simulink model "Copy_of_ModeStatAndRsp"  (R2018b)
settings: Solver=FixedStepDiscrete  StartTime=0.0  StopTime=10.0  FixedStep=0.01  RelTol=1e-3
undefined symbols (not defined in the file): c_RecvL, c_RecvLR, c_RecvR, IfVeSMSeStNumConfig, KeSMSbMdChime2Enable_Val, KeSMSbSRSPosNumConfig_Val, KeSMSuChmReqDurnTm_Val, KeSMSuChmReqIntlTm_Val, KeSMSuRspStatHldTm_Val, MdRspLocal1, MdTp1, ModeNum, PowerMode1, SrcReqTp1, srsconvert
libraries: RspLib x47, simulink x1
(part 3 of 8)

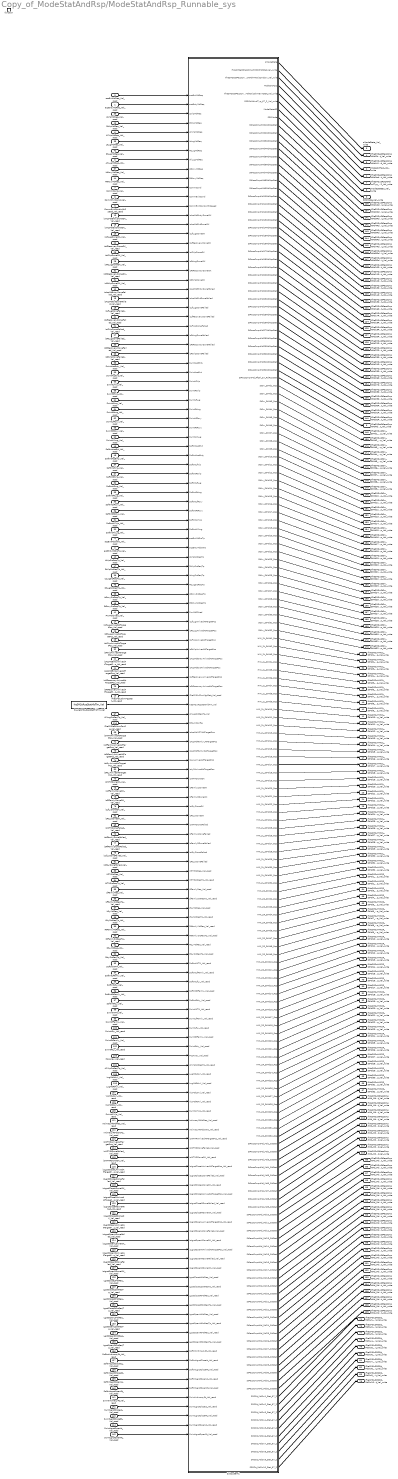
== system Copy_of_ModeStatAndRsp/ModeStatAndRsp_Runnable_sys ==
  acsEntyMdReq_Val_read : Inport
  acsEntyMdSrcTp_Val_read : Inport  Port=2
  acsExtMdReq_Val_read : Inport  Port=3
  acsExtMdSrcTp_Val_read : Inport  Port=4
  AllLugMdReq_Val_read : Inport  Port=5
  AllVipMdReq_Val_read : Inport  Port=6
  CommCond_Val_read : Inport  Port=7
  CommExitCond_Val_read : Inport  Port=8
  CommExitCondwithSpeed_Val_read : Inport  Port=9
  IfVeSMSuChmMgrStat_Val_read : Inport  Port=10
  isAcsMdEntryArrivedAtTargetPos_Val_read : Inport  Port=11
  isAcsMdEntryDoneFailed_Val_read : Inport  Port=12
  isAcsMdEntryDoneOK_Val_read : Inport  Port=13
  isAcsMdExtArrivedAtTargetPos_Val_read : Inport  Port=14
  isAcsMdExtDoneFailed_Val_read : Inport  Port=15
  isAcsMdExtDoneOK_Val_read : Inport  Port=16
  isLfLugArrivedAtTargetPos_Val_read : Inport  Port=17
  isLfLugDoneFailed_Val_read : Inport  Port=18
  isLfLugDoneOK_Val_read : Inport  Port=19
  isLfRecoveryArrivedAtTargetPos_Val_read : Inport  Port=20
  isLfRecoveryDoneFailed_Val_read : Inport  Port=21
  isLfRecoveryDoneOK_Val_read : Inport  Port=22
  isLfVipArrivedAtTargetPos_Val_read : Inport  Port=23
  isLfVipDoneFailed_Val_read : Inport  Port=24
  isLfVipDoneOK_Val_read : Inport  Port=25
  isRtLugArrivedAtTargetPos_Val_read : Inport  Port=26
  isRtLugDoneFailed_Val_read : Inport  Port=27
  isRtLugDoneOK_Val_read : Inport  Port=28
  isRtRecoveryArrivedAtTargetPos_Val_read : Inport  Port=29
  isRtRecoveryDoneFailed_Val_read : Inport  Port=30
  isRtRecoveryDoneOK_Val_read : Inport  Port=31
  isRtVipArrivedAtTargetPos_Val_read : Inport  Port=32
  isRtVipDoneFailed_Val_read : Inport  Port=33
  isRtVipDoneOK_Val_read : Inport  Port=34
  LtLugMdReq_Val_read : Inport  Port=35
  LtLugSrcReqTp_Val_read : Inport  Port=36
  LtRcvyMdReq_Val_read : Inport  Port=37
  LtRcvySrcReqTp_Val_read : Inport  Port=38
  LtVipMdReq_Val_read : Inport  Port=39
  LtVipSrcReqTp_Val_read : Inport  Port=40
  PwrMdChked_Val_read : Inport  Port=41
  RtLugMdReq_Val_read : Inport  Port=42
  RtLugSrcReqTp_Val_read : Inport  Port=43
  RtRcvyMdReq_Val_read : Inport  Port=44
  RtRcvySrcReqTp_Val_read : Inport  Port=45
  RtVipMdReq_Val_read : Inport  Port=46
  RtVipSrcReqTp_Val_read : Inport  Port=47
  SoftIntAcsEnty_Val_read : Inport  Port=48
  SoftIntAcsExt_Val_read : Inport  Port=49
  SoftIntAllLug_Val_read : Inport  Port=50
  SoftIntAllVip_Val_read : Inport  Port=51
  SoftIntLfLug_Val_read : Inport  Port=52
  SoftIntLfRcvy_Val_read : Inport  Port=53
  SoftIntLfVip_Val_read : Inport  Port=54
  SoftIntRtLug_Val_read : Inport  Port=55
  SoftIntRtRcvy_Val_read : Inport  Port=56
  SoftIntRtVip_Val_read : Inport  Port=57
  SwIntAcsEnty_Val_read : Inport  Port=58
  SwIntAcsExt_Val_read : Inport  Port=59
  SwIntAllLug_Val_read : Inport  Port=60
  SwIntLfLug_Val_read : Inport  Port=61
  SwIntLfRcvy_Val_read : Inport  Port=62
  SwIntLfVip_Val_read : Inport  Port=63
  SwIntRtLug_Val_read : Inport  Port=64
  SwIntRtRcvy_Val_read : Inport  Port=65
  SwIntRtVip_Val_read : Inport  Port=66
  AllLugSrcReqTp_Val_read : Inport  Port=67
  isINTMArrivedAtTargetPos_Val_read : Inport  Port=68
  isINTMDoneFailed_Val_read : Inport  Port=69
  isINTMDoneOK_Val_read : Inport  Port=70
  isLfFamlyArrivedAtTargetPos_Val_read : Inport  Port=71
  isLfFamlyDoneFailed_Val_read : Inport  Port=72
  isLfFamlyDoneOK_Val_read : Inport  Port=73
  isLfLyArrivedAtTargetPos_Val_read : Inport  Port=74
  isLfLyDoneFailed_Val_read : Inport  Port=75
  isLfLyDoneOK_Val_read : Inport  Port=76
  isRfFamlyDoneFailed_Val_read : Inport  Port=77
  isRfFamlyDoneOK_Val_read : Inport  Port=78
  isRtFamlyArrivedAtTargetPos_Val_read : Inport  Port=79
  isRtLyArrivedAtTargetPos_Val_read : Inport  Port=80
  isRtLyDoneFailed_Val_read : Inport  Port=81
  isRtLyDoneOK_Val_read : Inport  Port=82
  INTMMdReq_Val_read : Inport  Port=83
  INTMSrcReqTp_Val_read : Inport  Port=84
  LfFamlyReq_Val_read : Inport  Port=85
  LfFamlySrcReqTp_Val_read : Inport  Port=86
  LfLyMdReq_Val_read : Inport  Port=87
  LfLySrcReqTp_Val_read : Inport  Port=88
  RtFamlyMdReq_Val_read : Inport  Port=89
  RtFamlySrcReqTp_Val_read : Inport  Port=90
  RtLyMdReq_Val_read : Inport  Port=91
  RtLySrcReqTp_Val_read : Inport  Port=92
  SoftIntINTM_Val_read : Inport  Port=93
  SoftIntLfFamly_Val_read : Inport  Port=94
  SoftIntLfLy_Val_read : Inport  Port=95
  SoftIntRtFamly_Val_read : Inport  Port=96
  SoftIntRtLy_Val_read : Inport  Port=97
  SwIntINTM_Val_read : Inport  Port=98
  SwIntLfFamly_Val_read : Inport  Port=99
  SwIntLfLy_Val_read : Inport  Port=100
  SwIntRtFamly_Val_read : Inport  Port=101
  SwIntRtLy_Val_read : Inport  Port=102
  PosArray_Val_read : Inport  Port=103
  AllVipSrcReqTp_Val_read : Inport  Port=104
  LugMdLtAvl_Val_read : Inport  Port=105
  LugMdRtAvl_Val_read : Inport  Port=106
  VipMdLtAvl_Val_read : Inport  Port=107
  VipMdRtAvl_Val_read : Inport  Port=108
  SwIntAllVip_Val_read : Inport  Port=109
  IfVeSMSeStNumConfig_Val_read : Inport  Port=110
  IntimacyRtMdReq_Val_read : Inport  Port=111
  IntimacyRtMdSrcTp_Val_read : Inport  Port=112
  isINTMRArrivedAtTargetPos_Val_read : Inport  Port=113
  isINTMRDoneFailed_Val_read : Inport  Port=114
  isINTMRDoneOK_Val_read : Inport  Port=115
  isLgrstCloseLArrivedAtTargetPos_Val_read : Inport  Port=116
  isLgrstCloseLDoneFailed_Val_read : Inport  Port=117
  isLgrstCloseLDoneOK_Val_read : Inport  Port=118
  isLgrstCloseRArrivedAtTargetPos_Val_read : Inport  Port=119
  isLgrstCloseRDoneFailed_Val_read : Inport  Port=120
  isLgrstCloseRDoneOK_Val_read : Inport  Port=121
  isLgrstOpenLArrivedAtTargetPos_Val_read : Inport  Port=122
  isLgrstOpenLDoneFailed_Val_read : Inport  Port=123
  isLgrstOpenLDoneOK_Val_read : Inport  Port=124
  isLgrstOpenRArrivedAtTargetPos_Val_read : Inport  Port=125
  isLgrstOpenRDoneFailed_Val_read : Inport  Port=126
  isLgrstOpenRDoneOK_Val_read : Inport  Port=127
  LgrstCloseLtMdReq_Val_read : Inport  Port=128
  LgrstCloseLtSrcReqTp_Val_read : Inport  Port=129
  LgrstCloseRtMdReq_Val_read : Inport  Port=130
  LgrstCloseRtSrcReqTp_Val_read : Inport  Port=131
  LgrstOpenLtMdReq_Val_read : Inport  Port=132
  LgrstOpenLtSrcReqTp_Val_read : Inport  Port=133
  LgrstOpenRtMdReq_Val_read : Inport  Port=134
  LgrstOpenRtSrcReqTp_Val_read : Inport  Port=135
  SoftIntIntimacyRt_Val_read : Inport  Port=136
  SoftIntLgrstCloseLt_Val_read : Inport  Port=137
  SoftIntLgrstCloseRt_Val_read : Inport  Port=138
  SoftIntLgrstOpenLt_Val_read : Inport  Port=139
  SoftIntLgrstOpenRt_Val_read : Inport  Port=140
  SwIntIntimacyRt_Val_read : Inport  Port=141
  SwIntLgrstCloseLt_Val_read : Inport  Port=142
  SwIntLgrstCloseRt_Val_read : Inport  Port=143
  SwIntLgrstOpenLt_Val_read : Inport  Port=144
  SwIntLgrstOpenRt_Val_read : Inport  Port=145
  function : TriggerPort  TriggerType=function-call  VariantControl=(inherit)  SampleTimeType=periodic  SampleTime=-1
  PA_KeSMSuRspStatHldTm_Val : Constant  Value=KeSMSuRspStatHldTm_Val
  Subsystem1 : Subsystem
  IfVeSMSeStPassCmprtMdNoti2ChmEvntStat_Val_write : Outport
      settings: EnsureOutportIsVirtual=on
  ModeSrcTpLt_Val_write : Outport  Port=2
      settings: EnsureOutportIsVirtual=on
  oModeState_Val_write : Outport  Port=3
      settings: EnsureOutportIsVirtual=on
  IfVeSMSeStPassCmprtMdCrtMdStat_Val_write : Outport  Port=4
      settings: EnsureOutportIsVirtual=on
  IfVeSMSuStPassCmprtMdHMIDisCmd_Val_write : Outport  Port=5
      settings: EnsureOutportIsVirtual=on
  IfVeSMSeStPassCmprtMdRclRspStat_Val_write : Outport  Port=6
      settings: EnsureOutportIsVirtual=on
  IfVeSMSuSRSCrtMdIndTyp_67_2_Val_write : Outport  Port=7
      settings: EnsureOutportIsVirtual=on
  modestate32_Val_write : Outport  Port=8
      settings: EnsureOutportIsVirtual=on
  SRSMode_Val_write : Outport  Port=9
      settings: EnsureOutportIsVirtual=on
  IfVeSMSuHMI2L_StMd1_Rsp_Val_write : Outport  Port=10
      settings: EnsureOutportIsVirtual=on
  IfVeSMSuHMI2L_StMd10_Rsp_Val_write : Outport  Port=11
      settings: EnsureOutportIsVirtual=on
  IfVeSMSuHMI2L_StMd11_Rsp_Val_write : Outport  Port=12
      settings: EnsureOutportIsVirtual=on
  IfVeSMSuHMI2L_StMd12_Rsp_Val_write : Outport  Port=13
      settings: EnsureOutportIsVirtual=on
  IfVeSMSuHMI2L_StMd13_Rsp_Val_write : Outport  Port=14
      settings: EnsureOutportIsVirtual=on
  IfVeSMSuHMI2L_StMd14_Rsp_Val_write : Outport  Port=15
      settings: EnsureOutportIsVirtual=on
  IfVeSMSuHMI2L_StMd15_Rsp_Val_write : Outport  Port=16
      settings: EnsureOutportIsVirtual=on
  IfVeSMSuHMI2L_StMd16_Rsp_Val_write : Outport  Port=17
      settings: EnsureOutportIsVirtual=on
  IfVeSMSuHMI2L_StMd17_Rsp_Val_write : Outport  Port=18
      settings: EnsureOutportIsVirtual=on
  IfVeSMSuHMI2L_StMd18_Rsp_Val_write : Outport  Port=19
      settings: EnsureOutportIsVirtual=on
  IfVeSMSuHMI2L_StMd19_Rsp_Val_write : Outport  Port=20
      settings: EnsureOutportIsVirtual=on
  IfVeSMSuHMI2L_StMd2_Rsp_Val_write : Outport  Port=21
      settings: EnsureOutportIsVirtual=on
  IfVeSMSuHMI2L_StMd20_Rsp_Val_write : Outport  Port=22
      settings: EnsureOutportIsVirtual=on
  IfVeSMSuHMI2L_StMd21_Rsp_Val_write : Outport  Port=23
      settings: EnsureOutportIsVirtual=on
  IfVeSMSuHMI2L_StMd22_Rsp_Val_write : Outport  Port=24
      settings: EnsureOutportIsVirtual=on
  IfVeSMSuHMI2L_StMd23_Rsp_Val_write : Outport  Port=25
      settings: EnsureOutportIsVirtual=on
  IfVeSMSuHMI2L_StMd24_Rsp_Val_write : Outport  Port=26
      settings: EnsureOutportIsVirtual=on
  IfVeSMSuHMI2L_StMd25_Rsp_Val_write : Outport  Port=27
      settings: EnsureOutportIsVirtual=on
  IfVeSMSuHMI2L_StMd26_Rsp_Val_write : Outport  Port=28
      settings: EnsureOutportIsVirtual=on
  IfVeSMSuHMI2L_StMd27_Rsp_Val_write : Outport  Port=29
      settings: EnsureOutportIsVirtual=on
  IfVeSMSuHMI2L_StMd28_Rsp_Val_write : Outport  Port=30
      settings: EnsureOutportIsVirtual=on
  IfVeSMSuHMI2L_StMd29_Rsp_Val_write : Outport  Port=31
      settings: EnsureOutportIsVirtual=on
  IfVeSMSuHMI2L_StMd3_Rsp_Val_write : Outport  Port=32
      settings: EnsureOutportIsVirtual=on
  IfVeSMSuHMI2L_StMd30_Rsp_Val_write : Outport  Port=33
      settings: EnsureOutportIsVirtual=on
  IfVeSMSuHMI2L_StMd31_Rsp_Val_write : Outport  Port=34
      settings: EnsureOutportIsVirtual=on
  IfVeSMSuHMI2L_StMd32_Rsp_Val_write : Outport  Port=35
      settings: EnsureOutportIsVirtual=on
  IfVeSMSuHMI2L_StMd4_Rsp_Val_write : Outport  Port=36
      settings: EnsureOutportIsVirtual=on
  IfVeSMSuHMI2L_StMd5_Rsp_Val_write : Outport  Port=37
      settings: EnsureOutportIsVirtual=on
  IfVeSMSuHMI2L_StMd6_Rsp_Val_write : Outport  Port=38
      settings: EnsureOutportIsVirtual=on
  IfVeSMSuHMI2L_StMd7_Rsp_Val_write : Outport  Port=39
      settings: EnsureOutportIsVirtual=on
  IfVeSMSuHMI2L_StMd8_Rsp_Val_write : Outport  Port=40
      settings: EnsureOutportIsVirtual=on
  IfVeSMSuHMI2L_StMd9_Rsp_Val_write : Outport  Port=41
      settings: EnsureOutportIsVirtual=on
  IfVeSMSuHMI2R_StMd1_Rsp_Val_write : Outport  Port=42
      settings: EnsureOutportIsVirtual=on
  IfVeSMSuHMI2R_StMd10_Rsp_Val_write : Outport  Port=43
      settings: EnsureOutportIsVirtual=on
  IfVeSMSuHMI2R_StMd11_Rsp_Val_write : Outport  Port=44
      settings: EnsureOutportIsVirtual=on
  IfVeSMSuHMI2R_StMd12_Rsp_Val_write : Outport  Port=45
      settings: EnsureOutportIsVirtual=on
  IfVeSMSuHMI2R_StMd13_Rsp_Val_write : Outport  Port=46
      settings: EnsureOutportIsVirtual=on
  IfVeSMSuHMI2R_StMd14_Rsp_Val_write : Outport  Port=47
      settings: EnsureOutportIsVirtual=on
  IfVeSMSuHMI2R_StMd15_Rsp_Val_write : Outport  Port=48
      settings: EnsureOutportIsVirtual=on
  IfVeSMSuHMI2R_StMd16_Rsp_Val_write : Outport  Port=49
      settings: EnsureOutportIsVirtual=on
  IfVeSMSuHMI2R_StMd17_Rsp_Val_write : Outport  Port=50
      settings: EnsureOutportIsVirtual=on
  IfVeSMSuHMI2R_StMd18_Rsp_Val_write : Outport  Port=51
      settings: EnsureOutportIsVirtual=on
  IfVeSMSuHMI2R_StMd19_Rsp_Val_write : Outport  Port=52
      settings: EnsureOutportIsVirtual=on
  IfVeSMSuHMI2R_StMd2_Rsp_Val_write : Outport  Port=53
      settings: EnsureOutportIsVirtual=on
  IfVeSMSuHMI2R_StMd20_Rsp_Val_write : Outport  Port=54
      settings: EnsureOutportIsVirtual=on
  IfVeSMSuHMI2R_StMd21_Rsp_Val_write : Outport  Port=55
      settings: EnsureOutportIsVirtual=on
  IfVeSMSuHMI2R_StMd22_Rsp_Val_write : Outport  Port=56
      settings: EnsureOutportIsVirtual=on
  IfVeSMSuHMI2R_StMd23_Rsp_Val_write : Outport  Port=57
      settings: EnsureOutportIsVirtual=on
  IfVeSMSuHMI2R_StMd24_Rsp_Val_write : Outport  Port=58
      settings: EnsureOutportIsVirtual=on
  IfVeSMSuHMI2R_StMd25_Rsp_Val_write : Outport  Port=59
      settings: EnsureOutportIsVirtual=on
  IfVeSMSuHMI2R_StMd26_Rsp_Val_write : Outport  Port=60
      settings: EnsureOutportIsVirtual=on
  IfVeSMSuHMI2R_StMd27_Rsp_Val_write : Outport  Port=61
      settings: EnsureOutportIsVirtual=on
  IfVeSMSuHMI2R_StMd28_Rsp_Val_write : Outport  Port=62
      settings: EnsureOutportIsVirtual=on
  IfVeSMSuHMI2R_StMd29_Rsp_Val_write : Outport  Port=63
      settings: EnsureOutportIsVirtual=on
  IfVeSMSuHMI2R_StMd3_Rsp_Val_write : Outport  Port=64
      settings: EnsureOutportIsVirtual=on
  IfVeSMSuHMI2R_StMd30_Rsp_Val_write : Outport  Port=65
      settings: EnsureOutportIsVirtual=on
  IfVeSMSuHMI2R_StMd31_Rsp_Val_write : Outport  Port=66
      settings: EnsureOutportIsVirtual=on
  IfVeSMSuHMI2R_StMd32_Rsp_Val_write : Outport  Port=67
      settings: EnsureOutportIsVirtual=on
  IfVeSMSuHMI2R_StMd4_Rsp_Val_write : Outport  Port=68
      settings: EnsureOutportIsVirtual=on
  IfVeSMSuHMI2R_StMd5_Rsp_Val_write : Outport  Port=69
      settings: EnsureOutportIsVirtual=on
  IfVeSMSuHMI2R_StMd6_Rsp_Val_write : Outport  Port=70
      settings: EnsureOutportIsVirtual=on
  IfVeSMSuHMI2R_StMd7_Rsp_Val_write : Outport  Port=71
      settings: EnsureOutportIsVirtual=on
  IfVeSMSuHMI2R_StMd8_Rsp_Val_write : Outport  Port=72
      settings: EnsureOutportIsVirtual=on
  IfVeSMSuHMI2R_StMd9_Rsp_Val_write : Outport  Port=73
      settings: EnsureOutportIsVirtual=on
  IfVeSMSuSRSCrt_MdSw1_Stat_Val_write : Outport  Port=74
      settings: EnsureOutportIsVirtual=on
  IfVeSMSuSRSCrt_MdSw10_Stat_Val_write : Outport  Port=75
      settings: EnsureOutportIsVirtual=on
  IfVeSMSuSRSCrt_MdSw2_Stat_Val_write : Outport  Port=76
      settings: EnsureOutportIsVirtual=on
  IfVeSMSuSRSCrt_MdSw3_Stat_Val_write : Outport  Port=77
      settings: EnsureOutportIsVirtual=on
  IfVeSMSuSRSCrt_MdSw4_Stat_Val_write : Outport  Port=78
      settings: EnsureOutportIsVirtual=on
  IfVeSMSuSRSCrt_MdSw5_Stat_Val_write : Outport  Port=79
      settings: EnsureOutportIsVirtual=on
  IfVeSMSuSRSCrt_MdSw6_Stat_Val_write : Outport  Port=80
      settings: EnsureOutportIsVirtual=on
  IfVeSMSuSRSCrt_MdSw7_Stat_Val_write : Outport  Port=81
      settings: EnsureOutportIsVirtual=on
  IfVeSMSuSRSCrt_MdSw8_Stat_Val_write : Outport  Port=82
      settings: EnsureOutportIsVirtual=on
  IfVeSMSuSRSCrt_MdSw9_Stat_Val_write : Outport  Port=83
      settings: EnsureOutportIsVirtual=on
  IfVeSMSuStPassCmprtMd_Md1_CrtStat_Val_write : Outport  Port=84
      settings: EnsureOutportIsVirtual=on
  IfVeSMSuStPassCmprtMd_Md10_CrtStat_Val_write : Outport  Port=85
      settings: EnsureOutportIsVirtual=on
  IfVeSMSuStPassCmprtMd_Md11_CrtStat_Val_write : Outport  Port=86
      settings: EnsureOutportIsVirtual=on
  IfVeSMSuStPassCmprtMd_Md12_CrtStat_Val_write : Outport  Port=87
      settings: EnsureOutportIsVirtual=on
  IfVeSMSuStPassCmprtMd_Md13_CrtStat_Val_write : Outport  Port=88
      settings: EnsureOutportIsVirtual=on
  IfVeSMSuStPassCmprtMd_Md14_CrtStat_Val_write : Outport  Port=89
      settings: EnsureOutportIsVirtual=on
  IfVeSMSuStPassCmprtMd_Md15_CrtStat_Val_write : Outport  Port=90
      settings: EnsureOutportIsVirtual=on
  IfVeSMSuStPassCmprtMd_Md16_CrtStat_Val_write : Outport  Port=91
      settings: EnsureOutportIsVirtual=on
  IfVeSMSuStPassCmprtMd_Md17_CrtStat_Val_write : Outport  Port=92
      settings: EnsureOutportIsVirtual=on
  IfVeSMSuStPassCmprtMd_Md18_CrtStat_Val_write : Outport  Port=93
      settings: EnsureOutportIsVirtual=on
  IfVeSMSuStPassCmprtMd_Md19_CrtStat_Val_write : Outport  Port=94
      settings: EnsureOutportIsVirtual=on
  IfVeSMSuStPassCmprtMd_Md2_CrtStat_Val_write : Outport  Port=95
      settings: EnsureOutportIsVirtual=on
  IfVeSMSuStPassCmprtMd_Md20_CrtStat_Val_write : Outport  Port=96
      settings: EnsureOutportIsVirtual=on
  IfVeSMSuStPassCmprtMd_Md21_CrtStat_Val_write : Outport  Port=97
      settings: EnsureOutportIsVirtual=on
  IfVeSMSuStPassCmprtMd_Md22_CrtStat_Val_write : Outport  Port=98
      settings: EnsureOutportIsVirtual=on
  IfVeSMSuStPassCmprtMd_Md23_CrtStat_Val_write : Outport  Port=99
      settings: EnsureOutportIsVirtual=on
  IfVeSMSuStPassCmprtMd_Md24_CrtStat_Val_write : Outport  Port=100
      settings: EnsureOutportIsVirtual=on
  IfVeSMSuStPassCmprtMd_Md25_CrtStat_Val_write : Outport  Port=101
      settings: EnsureOutportIsVirtual=on
  IfVeSMSuStPassCmprtMd_Md26_CrtStat_Val_write : Outport  Port=102
      settings: EnsureOutportIsVirtual=on
  IfVeSMSuStPassCmprtMd_Md27_CrtStat_Val_write : Outport  Port=103
      settings: EnsureOutportIsVirtual=on
  IfVeSMSuStPassCmprtMd_Md28_CrtStat_Val_write : Outport  Port=104
      settings: EnsureOutportIsVirtual=on
  IfVeSMSuStPassCmprtMd_Md29_CrtStat_Val_write : Outport  Port=105
      settings: EnsureOutportIsVirtual=on
  IfVeSMSuStPassCmprtMd_Md3_CrtStat_Val_write : Outport  Port=106
      settings: EnsureOutportIsVirtual=on
  IfVeSMSuStPassCmprtMd_Md30_CrtStat_Val_write : Outport  Port=107
      settings: EnsureOutportIsVirtual=on
  IfVeSMSuStPassCmprtMd_Md31_CrtStat_Val_write : Outport  Port=108
      settings: EnsureOutportIsVirtual=on
  IfVeSMSuStPassCmprtMd_Md32_CrtStat_Val_write : Outport  Port=109
      settings: EnsureOutportIsVirtual=on
  IfVeSMSuStPassCmprtMd_Md4_CrtStat_Val_write : Outport  Port=110
      settings: EnsureOutportIsVirtual=on
  IfVeSMSuStPassCmprtMd_Md5_CrtStat_Val_write : Outport  Port=111
      settings: EnsureOutportIsVirtual=on
  IfVeSMSuStPassCmprtMd_Md6_CrtStat_Val_write : Outport  Port=112
      settings: EnsureOutportIsVirtual=on
  IfVeSMSuStPassCmprtMd_Md7_CrtStat_Val_write : Outport  Port=113
      settings: EnsureOutportIsVirtual=on
  IfVeSMSuStPassCmprtMd_Md8_CrtStat_Val_write : Outport  Port=114
      settings: EnsureOutportIsVirtual=on
  IfVeSMSuStPassCmprtMd_Md9_CrtStat_Val_write : Outport  Port=115
      settings: EnsureOutportIsVirtual=on
  IfVeSMSuStPassCmprtMd10RclRspStat_Val_write : Outport  Port=116
      settings: EnsureOutportIsVirtual=on
  IfVeSMSuStPassCmprtMd11RclRspStat_Val_write : Outport  Port=117
      settings: EnsureOutportIsVirtual=on
  IfVeSMSuStPassCmprtMd12RclRspStat_Val_write : Outport  Port=118
      settings: EnsureOutportIsVirtual=on
  IfVeSMSuStPassCmprtMd13RclRspStat_Val_write : Outport  Port=119
      settings: EnsureOutportIsVirtual=on
  IfVeSMSuStPassCmprtMd14RclRspStat_Val_write : Outport  Port=120
      settings: EnsureOutportIsVirtual=on
  IfVeSMSuStPassCmprtMd15RclRspStat_Val_write : Outport  Port=121
      settings: EnsureOutportIsVirtual=on
  IfVeSMSuStPassCmprtMd16RclRspStat_Val_write : Outport  Port=122
      settings: EnsureOutportIsVirtual=on
  IfVeSMSuStPassCmprtMd17RclRspStat_Val_write : Outport  Port=123
      settings: EnsureOutportIsVirtual=on
  IfVeSMSuStPassCmprtMd18RclRspStat_Val_write : Outport  Port=124
      settings: EnsureOutportIsVirtual=on
  IfVeSMSuStPassCmprtMd19RclRspStat_Val_write : Outport  Port=125
      settings: EnsureOutportIsVirtual=on
  IfVeSMSuStPassCmprtMd1RclRspStat_Val_write : Outport  Port=126
      settings: EnsureOutportIsVirtual=on
  IfVeSMSuStPassCmprtMd20RclRspStat_Val_write : Outport  Port=127
      settings: EnsureOutportIsVirtual=on
  IfVeSMSuStPassCmprtMd21RclRspStat_Val_write : Outport  Port=128
      settings: EnsureOutportIsVirtual=on
  IfVeSMSuStPassCmprtMd22RclRspStat_Val_write : Outport  Port=129
      settings: EnsureOutportIsVirtual=on
  IfVeSMSuStPassCmprtMd23RclRspStat_Val_write : Outport  Port=130
      settings: EnsureOutportIsVirtual=on
  IfVeSMSuStPassCmprtMd24RclRspStat_Val_write : Outport  Port=131
      settings: EnsureOutportIsVirtual=on
  IfVeSMSuStPassCmprtMd25RclRspStat_Val_write : Outport  Port=132
      settings: EnsureOutportIsVirtual=on
  IfVeSMSuStPassCmprtMd26RclRspStat_Val_write : Outport  Port=133
      settings: EnsureOutportIsVirtual=on
  IfVeSMSuStPassCmprtMd27RclRspStat_Val_write : Outport  Port=134
      settings: EnsureOutportIsVirtual=on
  IfVeSMSuStPassCmprtMd28RclRspStat_Val_write : Outport  Port=135
      settings: EnsureOutportIsVirtual=on
  IfVeSMSuStPassCmprtMd29RclRspStat_Val_write : Outport  Port=136
      settings: EnsureOutportIsVirtual=on
  IfVeSMSuStPassCmprtMd2RclRspStat_Val_write : Outport  Port=137
      settings: EnsureOutportIsVirtual=on
  IfVeSMSuStPassCmprtMd30RclRspStat_Val_write : Outport  Port=138
      settings: EnsureOutportIsVirtual=on
  IfVeSMSuStPassCmprtMd31RclRspStat_Val_write : Outport  Port=139
      settings: EnsureOutportIsVirtual=on
  IfVeSMSuStPassCmprtMd32RclRspStat_Val_write : Outport  Port=140
      settings: EnsureOutportIsVirtual=on
  IfVeSMSuStPassCmprtMd3RclRspStat_Val_write : Outport  Port=141
      settings: EnsureOutportIsVirtual=on
  IfVeSMSuStPassCmprtMd4RclRspStat_Val_write : Outport  Port=142
      settings: EnsureOutportIsVirtual=on
  IfVeSMSuStPassCmprtMd5RclRspStat_Val_write : Outport  Port=143
      settings: EnsureOutportIsVirtual=on
  IfVeSMSuStPassCmprtMd6RclRspStat_Val_write : Outport  Port=144
      settings: EnsureOutportIsVirtual=on
  IfVeSMSuStPassCmprtMd7RclRspStat_Val_write : Outport  Port=145
      settings: EnsureOutportIsVirtual=on
  IfVeSMSuStPassCmprtMd8RclRspStat_Val_write : Outport  Port=146
      settings: EnsureOutportIsVirtual=on
  IfVeSMSuStPassCmprtMd9RclRspStat_Val_write : Outport  Port=147
      settings: EnsureOutportIsVirtual=on
  IfVeSMSuStSrv_StMd1_Rsp_Val_write : Outport  Port=148
      settings: EnsureOutportIsVirtual=on
  IfVeSMSuStSrv_StMd10_Rsp_Val_write : Outport  Port=149
      settings: EnsureOutportIsVirtual=on
  IfVeSMSuStSrv_StMd11_Rsp_Val_write : Outport  Port=150
      settings: EnsureOutportIsVirtual=on
  IfVeSMSuStSrv_StMd12_Rsp_Val_write : Outport  Port=151
      settings: EnsureOutportIsVirtual=on
  IfVeSMSuStSrv_StMd13_Rsp_Val_write : Outport  Port=152
      settings: EnsureOutportIsVirtual=on
  IfVeSMSuStSrv_StMd14_Rsp_Val_write : Outport  Port=153
      settings: EnsureOutportIsVirtual=on
  IfVeSMSuStSrv_StMd15_Rsp_Val_write : Outport  Port=154
      settings: EnsureOutportIsVirtual=on
  IfVeSMSuStSrv_StMd16_Rsp_Val_write : Outport  Port=155
      settings: EnsureOutportIsVirtual=on
  IfVeSMSuStSrv_StMd17_Rsp_Val_write : Outport  Port=156
      settings: EnsureOutportIsVirtual=on
  IfVeSMSuStSrv_StMd18_Rsp_Val_write : Outport  Port=157
      settings: EnsureOutportIsVirtual=on
  IfVeSMSuStSrv_StMd19_Rsp_Val_write : Outport  Port=158
      settings: EnsureOutportIsVirtual=on
  IfVeSMSuStSrv_StMd2_Rsp_Val_write : Outport  Port=159
      settings: EnsureOutportIsVirtual=on
  IfVeSMSuStSrv_StMd20_Rsp_Val_write : Outport  Port=160
      settings: EnsureOutportIsVirtual=on
  IfVeSMSuStSrv_StMd21_Rsp_Val_write : Outport  Port=161
      settings: EnsureOutportIsVirtual=on
  IfVeSMSuStSrv_StMd22_Rsp_Val_write : Outport  Port=162
      settings: EnsureOutportIsVirtual=on
  IfVeSMSuStSrv_StMd23_Rsp_Val_write : Outport  Port=163
      settings: EnsureOutportIsVirtual=on
  IfVeSMSuStSrv_StMd24_Rsp_Val_write : Outport  Port=164
      settings: EnsureOutportIsVirtual=on
  IfVeSMSuStSrv_StMd25_Rsp_Val_write : Outport  Port=165
      settings: EnsureOutportIsVirtual=on
  IfVeSMSuStSrv_StMd26_Rsp_Val_write : Outport  Port=166
      settings: EnsureOutportIsVirtual=on
  IfVeSMSuStSrv_StMd27_Rsp_Val_write : Outport  Port=167
      settings: EnsureOutportIsVirtual=on
  IfVeSMSuStSrv_StMd28_Rsp_Val_write : Outport  Port=168
      settings: EnsureOutportIsVirtual=on
  IfVeSMSuStSrv_StMd29_Rsp_Val_write : Outport  Port=169
      settings: EnsureOutportIsVirtual=on
  IfVeSMSuStSrv_StMd3_Rsp_Val_write : Outport  Port=170
      settings: EnsureOutportIsVirtual=on
  IfVeSMSuStSrv_StMd30_Rsp_Val_write : Outport  Port=171
      settings: EnsureOutportIsVirtual=on
  IfVeSMSuStSrv_StMd31_Rsp_Val_write : Outport  Port=172
      settings: EnsureOutportIsVirtual=on
  IfVeSMSuStSrv_StMd32_Rsp_Val_write : Outport  Port=173
      settings: EnsureOutportIsVirtual=on
  IfVeSMSuStSrv_StMd4_Rsp_Val_write : Outport  Port=174
      settings: EnsureOutportIsVirtual=on
  IfVeSMSuStSrv_StMd5_Rsp_Val_write : Outport  Port=175
      settings: EnsureOutportIsVirtual=on
  IfVeSMSuStSrv_StMd6_Rsp_Val_write : Outport  Port=176
      settings: EnsureOutportIsVirtual=on
  IfVeSMSuStSrv_StMd7_Rsp_Val_write : Outport  Port=177
      settings: EnsureOutportIsVirtual=on
  IfVeSMSuStSrv_StMd8_Rsp_Val_write : Outport  Port=178
      settings: EnsureOutportIsVirtual=on
  IfVeSMSuStSrv_StMd9_Rsp_Val_write : Outport  Port=179
      settings: EnsureOutportIsVirtual=on
  wires:
  acsEntyMdSrcTp_Val_read/1 -> Subsystem1/50(acsEntyMdSrcTp)
  acsExtMdReq_Val_read/1 -> Subsystem1/1(acsExtMdReq)
  acsExtMdSrcTp_Val_read/1 -> Subsystem1/49(acsExtMdSrcTp)
  AllLugMdReq_Val_read/1 -> Subsystem1/8(AllLugMdReq)
  AllVipMdReq_Val_read/1 -> Subsystem1/5(AllVipMdReq)
  CommCond_Val_read/1 -> Subsystem1/11(CommCond)
  CommExitCond_Val_read/1 -> Subsystem1/12(CommExitCond)
  CommExitCondwithSpeed_Val_read/1 -> Subsystem1/13(CommExitCondwithSpeed)
  IfVeSMSuChmMgrStat_Val_read/1 -> Subsystem1/66(IfVeSMSuChmMgrStat_Val_read)
  isAcsMdEntryArrivedAtTargetPos_Val_read/1 -> Subsystem1/62(isAcsMdEntryArrivedAtTargetPos)
  isAcsMdEntryDoneFailed_Val_read/1 -> Subsystem1/22(isAcsMdEntryDoneFailed)
  isAcsMdEntryDoneOK_Val_read/1 -> Subsystem1/14(isAcsMdEntryDoneOK)
  isAcsMdExtArrivedAtTargetPos_Val_read/1 -> Subsystem1/63(isAcsMdExtArrivedAtTargetPos)
  isAcsMdExtDoneFailed_Val_read/1 -> Subsystem1/23(isAcsMdExtDoneFailed)
  isAcsMdExtDoneOK_Val_read/1 -> Subsystem1/15(isAcsMdExtDoneOK)
  isLfLugDoneFailed_Val_read/1 -> Subsystem1/24(isLfLugDoneFailed)
  isLfLugDoneOK_Val_read/1 -> Subsystem1/16(isLfLugDoneOK)
  isLfRecoveryArrivedAtTargetPos_Val_read/1 -> Subsystem1/64(isLfRecoveryArrivedAtTargetPos)
  isLfRecoveryDoneFailed_Val_read/1 -> Subsystem1/25(isLfRecoveryDoneFailed)
  isLfRecoveryDoneOK_Val_read/1 -> Subsystem1/17(isLfRecoveryDoneOK)
  isLfVipArrivedAtTargetPos_Val_read/1 -> Subsystem1/60(isLfVipArrivedAtTargetPos)
  isLfVipDoneFailed_Val_read/1 -> Subsystem1/26(isLfVipDoneFailed)
  isLfVipDoneOK_Val_read/1 -> Subsystem1/18(isLfVipDoneOK)
  isRtLugArrivedAtTargetPos_Val_read/1 -> Subsystem1/59(isRtLugArrivedAtTargetPos)
  isRtLugDoneFailed_Val_read/1 -> Subsystem1/27(isRtLugDoneFailed)
  isRtLugDoneOK_Val_read/1 -> Subsystem1/19(isRtLugDoneOK)
  isRtRecoveryArrivedAtTargetPos_Val_read/1 -> Subsystem1/65(isRtRecoveryArrivedAtTargetPos)
  isRtRecoveryDoneFailed_Val_read/1 -> Subsystem1/28(isRtRecoveryDoneFailed)
  isRtRecoveryDoneOK_Val_read/1 -> Subsystem1/20(isRtRecoveryDoneOK)
  isRtVipArrivedAtTargetPos_Val_read/1 -> Subsystem1/61(isRtVipArrivedAtTargetPos)
  isRtVipDoneFailed_Val_read/1 -> Subsystem1/29(isRtVipDoneFailed)
  isRtVipDoneOK_Val_read/1 -> Subsystem1/21(isRtVipDoneOK)
  LtLugMdReq_Val_read/1 -> Subsystem1/6(LtLugMdReq)
  LtLugSrcReqTp_Val_read/1 -> Subsystem1/53(LtLugSrcReqTp)
  LtRcvyMdReq_Val_read/1 -> Subsystem1/9(LtRcvyMdReq)
  LtRcvySrcReqTp_Val_read/1 -> Subsystem1/55(LtRcvySrcReqTp)
  LtVipMdReq_Val_read/1 -> Subsystem1/3(LtVipMdReq)
  LtVipSrcReqTp_Val_read/1 -> Subsystem1/51(LtVipSrcReqTp)
  PwrMdChked_Val_read/1 -> Subsystem1/57(PwrMdChked)
  RtLugMdReq_Val_read/1 -> Subsystem1/7(RtLugMdReq)
  RtLugSrcReqTp_Val_read/1 -> Subsystem1/54(RtLugSrcReqTp)
  RtRcvyMdReq_Val_read/1 -> Subsystem1/10(RtRcvyMdReq)
  RtRcvySrcReqTp_Val_read/1 -> Subsystem1/56(RtRcvySrcReqTp)
  RtVipMdReq_Val_read/1 -> Subsystem1/4(RtVipMdReq)
  RtVipSrcReqTp_Val_read/1 -> Subsystem1/52(RtVipSrcReqTp)
  SoftIntAcsEnty_Val_read/1 -> Subsystem1/40(SoftIntAcsEnty)
  SoftIntAcsExt_Val_read/1 -> Subsystem1/39(SoftIntAcsExt)
  SoftIntAllLug_Val_read/1 -> Subsystem1/48(SoftIntAllLug)
  SoftIntAllVip_Val_read/1 -> Subsystem1/47(SoftIntAllVip)
  SoftIntLfLug_Val_read/1 -> Subsystem1/43(SoftIntLfLug)
  SoftIntLfRcvy_Val_read/1 -> Subsystem1/45(SoftIntLfRcvy)
  SoftIntLfVip_Val_read/1 -> Subsystem1/41(SoftIntLfVip)
  SoftIntRtLug_Val_read/1 -> Subsystem1/44(SoftIntRtLug)
  SoftIntRtRcvy_Val_read/1 -> Subsystem1/46(SoftIntRtRcvy)
  SoftIntRtVip_Val_read/1 -> Subsystem1/42(SoftIntRtVip)
  SwIntAcsEnty_Val_read/1 -> Subsystem1/30(SwIntAcsEnty)
  SwIntAcsExt_Val_read/1 -> Subsystem1/31(SwIntAcsExt)
  SwIntAllLug_Val_read/1 -> Subsystem1/38(SwIntAllLug)
  SwIntLfLug_Val_read/1 -> Subsystem1/34(SwIntLfLug)
  SwIntLfRcvy_Val_read/1 -> Subsystem1/36(SwIntLfRcvy)
  SwIntLfVip_Val_read/1 -> Subsystem1/32(SwIntLfVip)
  SwIntRtLug_Val_read/1 -> Subsystem1/35(SwIntRtLug)
  SwIntRtRcvy_Val_read/1 -> Subsystem1/37(SwIntRtRcvy)
  SwIntRtVip_Val_read/1 -> Subsystem1/33(SwIntRtVip)
  PA_KeSMSuRspStatHldTm_Val/1 -> Subsystem1/67(KeSMSuRspStatHldTm_Val)
  Subsystem1/5(IfVeSMSeStPassCmprtMdNoti2ChmEvntStat_Val_write) -> IfVeSMSeStPassCmprtMdNoti2ChmEvntStat_Val_write/1
  Subsystem1/4(ModeSrcTpLt) -> ModeSrcTpLt_Val_write/1
  Subsystem1/1(oModeState) -> oModeState_Val_write/1
  Subsystem1/3(IfVeSMSeStPassCmprtMdHMIDisCmdSrv_Val_write) -> IfVeSMSuStPassCmprtMdHMIDisCmd_Val_write/1
  Subsystem1/2(IfVeSMSeStPassCmprtMdCrtMdStat_Val_write) -> IfVeSMSeStPassCmprtMdCrtMdStat_Val_write/1
  Subsystem1/41(StPassCmprtMd_RfCtrl_Sw_RclRspStat) -> IfVeSMSeStPassCmprtMdRclRspStat_Val_write/1
  acsEntyMdReq_Val_read/1 -> Subsystem1/2(acsEntyMdReq)
  isLfLugArrivedAtTargetPos_Val_read/1 -> Subsystem1/58(isLfLugArrivedAtTargetPos)
  AllLugSrcReqTp_Val_read/1 -> Subsystem1/68(AllLugSrcReqTp_Val)
  Subsystem1/6(SRSCrtMdIndTyp_67_2_Val_write) -> IfVeSMSuSRSCrtMdIndTyp_67_2_Val_write/1
  Subsystem1/7(ModeState32) -> modestate32_Val_write/1
  Subsystem1/8(SRSMode) -> SRSMode_Val_write/1
  IfVeSMSeStNumConfig_Val_read/1 -> Subsystem1/69(StNumConfig)
  Subsystem1/76(HMI_2L_StMd3_Rsp) -> IfVeSMSuHMI2L_StMd3_Rsp_Val_write/1
  Subsystem1/77(HMI_2L_StMd4_Rsp) -> IfVeSMSuHMI2L_StMd4_Rsp_Val_write/1
  Subsystem1/78(HMI_2L_StMd5_Rsp) -> IfVeSMSuHMI2L_StMd5_Rsp_Val_write/1
  Subsystem1/79(HMI_2L_StMd6_Rsp) -> IfVeSMSuHMI2L_StMd6_Rsp_Val_write/1
  Subsystem1/80(HMI_2L_StMd7_Rsp) -> IfVeSMSuHMI2L_StMd7_Rsp_Val_write/1
  Subsystem1/81(HMI_2L_StMd8_Rsp) -> IfVeSMSuHMI2L_StMd8_Rsp_Val_write/1
  Subsystem1/82(HMI_2L_StMd9_Rsp) -> IfVeSMSuHMI2L_StMd9_Rsp_Val_write/1
  Subsystem1/94(HMI_2L_StMd21_Rsp) -> IfVeSMSuHMI2L_StMd21_Rsp_Val_write/1
  Subsystem1/95(HMI_2L_StMd22_Rsp) -> IfVeSMSuHMI2L_StMd22_Rsp_Val_write/1
  Subsystem1/96(HMI_2L_StMd23_Rsp) -> IfVeSMSuHMI2L_StMd23_Rsp_Val_write/1
  Subsystem1/97(HMI_2L_StMd24_Rsp) -> IfVeSMSuHMI2L_StMd24_Rsp_Val_write/1
  Subsystem1/98(HMI_2L_StMd25_Rsp) -> IfVeSMSuHMI2L_StMd25_Rsp_Val_write/1
  Subsystem1/99(HMI_2L_StMd26_Rsp) -> IfVeSMSuHMI2L_StMd26_Rsp_Val_write/1
  Subsystem1/100(HMI_2L_StMd27_Rsp) -> IfVeSMSuHMI2L_StMd27_Rsp_Val_write/1
  Subsystem1/101(HMI_2L_StMd28_Rsp) -> IfVeSMSuHMI2L_StMd28_Rsp_Val_write/1
  Subsystem1/104(HMI_2L_StMd31_Rsp) -> IfVeSMSuHMI2L_StMd31_Rsp_Val_write/1
  Subsystem1/105(HMI_2L_StMd32_Rsp) -> IfVeSMSuHMI2L_StMd32_Rsp_Val_write/1
  Subsystem1/74(HMI_2L_StMd1_Rsp) -> IfVeSMSuHMI2L_StMd1_Rsp_Val_write/1
  Subsystem1/83(HMI_2L_StMd10_Rsp) -> IfVeSMSuHMI2L_StMd10_Rsp_Val_write/1
  Subsystem1/84(HMI_2L_StMd11_Rsp) -> IfVeSMSuHMI2L_StMd11_Rsp_Val_write/1
  Subsystem1/85(HMI_2L_StMd12_Rsp) -> IfVeSMSuHMI2L_StMd12_Rsp_Val_write/1
  Subsystem1/86(HMI_2L_StMd13_Rsp) -> IfVeSMSuHMI2L_StMd13_Rsp_Val_write/1
  Subsystem1/87(HMI_2L_StMd14_Rsp) -> IfVeSMSuHMI2L_StMd14_Rsp_Val_write/1
  Subsystem1/88(HMI_2L_StMd15_Rsp) -> IfVeSMSuHMI2L_StMd15_Rsp_Val_write/1
  Subsystem1/89(HMI_2L_StMd16_Rsp) -> IfVeSMSuHMI2L_StMd16_Rsp_Val_write/1
  Subsystem1/90(HMI_2L_StMd17_Rsp) -> IfVeSMSuHMI2L_StMd17_Rsp_Val_write/1
  Subsystem1/91(HMI_2L_StMd18_Rsp) -> IfVeSMSuHMI2L_StMd18_Rsp_Val_write/1
  Subsystem1/92(HMI_2L_StMd19_Rsp) -> IfVeSMSuHMI2L_StMd19_Rsp_Val_write/1
  Subsystem1/75(HMI_2L_StMd2_Rsp) -> IfVeSMSuHMI2L_StMd2_Rsp_Val_write/1
  Subsystem1/93(HMI_2L_StMd20_Rsp) -> IfVeSMSuHMI2L_StMd20_Rsp_Val_write/1
  Subsystem1/102(HMI_2L_StMd29_Rsp) -> IfVeSMSuHMI2L_StMd29_Rsp_Val_write/1
  Subsystem1/103(HMI_2L_StMd30_Rsp) -> IfVeSMSuHMI2L_StMd30_Rsp_Val_write/1
  Subsystem1/106(HMI_2R_StMd1_Rsp) -> IfVeSMSuHMI2R_StMd1_Rsp_Val_write/1
  Subsystem1/107(HMI_2R_StMd2_Rsp) -> IfVeSMSuHMI2R_StMd2_Rsp_Val_write/1
  Subsystem1/115(HMI_2R_StMd10_Rsp) -> IfVeSMSuHMI2R_StMd10_Rsp_Val_write/1
  Subsystem1/116(HMI_2R_StMd11_Rsp) -> IfVeSMSuHMI2R_StMd11_Rsp_Val_write/1
  Subsystem1/117(HMI_2R_StMd12_Rsp) -> IfVeSMSuHMI2R_StMd12_Rsp_Val_write/1
  Subsystem1/118(HMI_2R_StMd13_Rsp) -> IfVeSMSuHMI2R_StMd13_Rsp_Val_write/1
  Subsystem1/119(HMI_2R_StMd14_Rsp) -> IfVeSMSuHMI2R_StMd14_Rsp_Val_write/1
  Subsystem1/120(HMI_2R_StMd15_Rsp) -> IfVeSMSuHMI2R_StMd15_Rsp_Val_write/1
  Subsystem1/121(HMI_2R_StMd16_Rsp) -> IfVeSMSuHMI2R_StMd16_Rsp_Val_write/1
  Subsystem1/122(HMI_2R_StMd17_Rsp) -> IfVeSMSuHMI2R_StMd17_Rsp_Val_write/1
  Subsystem1/123(HMI_2R_StMd18_Rsp) -> IfVeSMSuHMI2R_StMd18_Rsp_Val_write/1
  Subsystem1/124(HMI_2R_StMd19_Rsp) -> IfVeSMSuHMI2R_StMd19_Rsp_Val_write/1
  Subsystem1/125(HMI_2R_StMd20_Rsp) -> IfVeSMSuHMI2R_StMd20_Rsp_Val_write/1
  Subsystem1/126(HMI_2R_StMd21_Rsp) -> IfVeSMSuHMI2R_StMd21_Rsp_Val_write/1
  Subsystem1/127(HMI_2R_StMd22_Rsp) -> IfVeSMSuHMI2R_StMd22_Rsp_Val_write/1
  Subsystem1/128(HMI_2R_StMd23_Rsp) -> IfVeSMSuHMI2R_StMd23_Rsp_Val_write/1
  Subsystem1/129(HMI_2R_StMd24_Rsp) -> IfVeSMSuHMI2R_StMd24_Rsp_Val_write/1
  Subsystem1/130(HMI_2R_StMd25_Rsp) -> IfVeSMSuHMI2R_StMd25_Rsp_Val_write/1
  Subsystem1/131(HMI_2R_StMd26_Rsp) -> IfVeSMSuHMI2R_StMd26_Rsp_Val_write/1
  Subsystem1/132(HMI_2R_StMd27_Rsp) -> IfVeSMSuHMI2R_StMd27_Rsp_Val_write/1
  Subsystem1/133(HMI_2R_StMd28_Rsp) -> IfVeSMSuHMI2R_StMd28_Rsp_Val_write/1
  Subsystem1/134(HMI_2R_StMd29_Rsp) -> IfVeSMSuHMI2R_StMd29_Rsp_Val_write/1
  Subsystem1/135(HMI_2R_StMd30_Rsp) -> IfVeSMSuHMI2R_StMd30_Rsp_Val_write/1
  Subsystem1/136(HMI_2R_StMd31_Rsp) -> IfVeSMSuHMI2R_StMd31_Rsp_Val_write/1
  Subsystem1/137(HMI_2R_StMd32_Rsp) -> IfVeSMSuHMI2R_StMd32_Rsp_Val_write/1
  Subsystem1/108(HMI_2R_StMd3_Rsp) -> IfVeSMSuHMI2R_StMd3_Rsp_Val_write/1
  Subsystem1/109(HMI_2R_StMd4_Rsp) -> IfVeSMSuHMI2R_StMd4_Rsp_Val_write/1
  Subsystem1/110(HMI_2R_StMd5_Rsp) -> IfVeSMSuHMI2R_StMd5_Rsp_Val_write/1
  Subsystem1/111(HMI_2R_StMd6_Rsp) -> IfVeSMSuHMI2R_StMd6_Rsp_Val_write/1
  Subsystem1/112(HMI_2R_StMd7_Rsp) -> IfVeSMSuHMI2R_StMd7_Rsp_Val_write/1
  Subsystem1/113(HMI_2R_StMd8_Rsp) -> IfVeSMSuHMI2R_StMd8_Rsp_Val_write/1
  Subsystem1/114(HMI_2R_StMd9_Rsp) -> IfVeSMSuHMI2R_StMd9_Rsp_Val_write/1
  Subsystem1/170(SRSCrt_MdSw1_Stat_67_2) -> IfVeSMSuSRSCrt_MdSw1_Stat_Val_write/1
  Subsystem1/171(SRSCrt_MdSw2_Stat_67_2) -> IfVeSMSuSRSCrt_MdSw2_Stat_Val_write/1
  Subsystem1/172(SRSCrt_MdSw3_Stat_67_2) -> IfVeSMSuSRSCrt_MdSw3_Stat_Val_write/1
  Subsystem1/173(SRSCrt_MdSw4_Stat_67_2) -> IfVeSMSuSRSCrt_MdSw4_Stat_Val_write/1
  Subsystem1/174(SRSCrt_MdSw5_Stat_67_2) -> IfVeSMSuSRSCrt_MdSw5_Stat_Val_write/1
  Subsystem1/175(SRSCrt_MdSw6_Stat_67_2) -> IfVeSMSuSRSCrt_MdSw6_Stat_Val_write/1
  Subsystem1/176(SRSCrt_MdSw7_Stat_67_2) -> IfVeSMSuSRSCrt_MdSw7_Stat_Val_write/1
  Subsystem1/177(SRSCrt_MdSw8_Stat_67_2) -> IfVeSMSuSRSCrt_MdSw8_Stat_Val_write/1
  Subsystem1/178(SRSCrt_MdSw9_Stat_67_2) -> IfVeSMSuSRSCrt_MdSw9_Stat_Val_write/1
  Subsystem1/179(SRSCrt_MdSw10_Stat_67_2) -> IfVeSMSuSRSCrt_MdSw10_Stat_Val_write/1
  Subsystem1/138(StPassCmprtMd_Md1_CrtStat) -> IfVeSMSuStPassCmprtMd_Md1_CrtStat_Val_write/1
  Subsystem1/147(StPassCmprtMd_Md10_CrtStat) -> IfVeSMSuStPassCmprtMd_Md10_CrtStat_Val_write/1
  Subsystem1/148(StPassCmprtMd_Md11_CrtStat) -> IfVeSMSuStPassCmprtMd_Md11_CrtStat_Val_write/1
  Subsystem1/149(StPassCmprtMd_Md12_CrtStat) -> IfVeSMSuStPassCmprtMd_Md12_CrtStat_Val_write/1
  Subsystem1/150(StPassCmprtMd_Md13_CrtStat) -> IfVeSMSuStPassCmprtMd_Md13_CrtStat_Val_write/1
  Subsystem1/151(StPassCmprtMd_Md14_CrtStat) -> IfVeSMSuStPassCmprtMd_Md14_CrtStat_Val_write/1
  Subsystem1/152(StPassCmprtMd_Md15_CrtStat) -> IfVeSMSuStPassCmprtMd_Md15_CrtStat_Val_write/1
  Subsystem1/153(StPassCmprtMd_Md16_CrtStat) -> IfVeSMSuStPassCmprtMd_Md16_CrtStat_Val_write/1
  Subsystem1/154(StPassCmprtMd_Md17_CrtStat) -> IfVeSMSuStPassCmprtMd_Md17_CrtStat_Val_write/1
  Subsystem1/155(StPassCmprtMd_Md18_CrtStat) -> IfVeSMSuStPassCmprtMd_Md18_CrtStat_Val_write/1
  Subsystem1/156(StPassCmprtMd_Md19_CrtStat) -> IfVeSMSuStPassCmprtMd_Md19_CrtStat_Val_write/1
  Subsystem1/157(StPassCmprtMd_Md20_CrtStat) -> IfVeSMSuStPassCmprtMd_Md20_CrtStat_Val_write/1
  Subsystem1/158(StPassCmprtMd_Md21_CrtStat) -> IfVeSMSuStPassCmprtMd_Md21_CrtStat_Val_write/1
  Subsystem1/159(StPassCmprtMd_Md22_CrtStat) -> IfVeSMSuStPassCmprtMd_Md22_CrtStat_Val_write/1
  Subsystem1/160(StPassCmprtMd_Md23_CrtStat) -> IfVeSMSuStPassCmprtMd_Md23_CrtStat_Val_write/1
  Subsystem1/161(StPassCmprtMd_Md24_CrtStat) -> IfVeSMSuStPassCmprtMd_Md24_CrtStat_Val_write/1
  Subsystem1/162(StPassCmprtMd_Md25_CrtStat) -> IfVeSMSuStPassCmprtMd_Md25_CrtStat_Val_write/1
  Subsystem1/163(StPassCmprtMd_Md26_CrtStat) -> IfVeSMSuStPassCmprtMd_Md26_CrtStat_Val_write/1
  Subsystem1/164(StPassCmprtMd_Md27_CrtStat) -> IfVeSMSuStPassCmprtMd_Md27_CrtStat_Val_write/1
  Subsystem1/165(StPassCmprtMd_Md28_CrtStat) -> IfVeSMSuStPassCmprtMd_Md28_CrtStat_Val_write/1
  Subsystem1/166(StPassCmprtMd_Md29_CrtStat) -> IfVeSMSuStPassCmprtMd_Md29_CrtStat_Val_write/1
  Subsystem1/167(StPassCmprtMd_Md30_CrtStat) -> IfVeSMSuStPassCmprtMd_Md30_CrtStat_Val_write/1
  Subsystem1/168(StPassCmprtMd_Md31_CrtStat) -> IfVeSMSuStPassCmprtMd_Md31_CrtStat_Val_write/1
  Subsystem1/169(StPassCmprtMd_Md32_CrtStat) -> IfVeSMSuStPassCmprtMd_Md32_CrtStat_Val_write/1
  Subsystem1/139(StPassCmprtMd_Md2_CrtStat) -> IfVeSMSuStPassCmprtMd_Md2_CrtStat_Val_write/1
  Subsystem1/140(StPassCmprtMd_Md3_CrtStat) -> IfVeSMSuStPassCmprtMd_Md3_CrtStat_Val_write/1
  Subsystem1/141(StPassCmprtMd_Md4_CrtStat) -> IfVeSMSuStPassCmprtMd_Md4_CrtStat_Val_write/1
  Subsystem1/142(StPassCmprtMd_Md5_CrtStat) -> IfVeSMSuStPassCmprtMd_Md5_CrtStat_Val_write/1
  Subsystem1/143(StPassCmprtMd_Md6_CrtStat) -> IfVeSMSuStPassCmprtMd_Md6_CrtStat_Val_write/1
  Subsystem1/144(StPassCmprtMd_Md7_CrtStat) -> IfVeSMSuStPassCmprtMd_Md7_CrtStat_Val_write/1
  Subsystem1/145(StPassCmprtMd_Md8_CrtStat) -> IfVeSMSuStPassCmprtMd_Md8_CrtStat_Val_write/1
  Subsystem1/146(StPassCmprtMd_Md9_CrtStat) -> IfVeSMSuStPassCmprtMd_Md9_CrtStat_Val_write/1
  Subsystem1/40(StPassCmprtMd32RclRspStat) -> IfVeSMSuStPassCmprtMd32RclRspStat_Val_write/1
  Subsystem1/39(StPassCmprtMd31RclRspStat) -> IfVeSMSuStPassCmprtMd31RclRspStat_Val_write/1
  Subsystem1/38(StPassCmprtMd30RclRspStat) -> IfVeSMSuStPassCmprtMd30RclRspStat_Val_write/1
  Subsystem1/37(StPassCmprtMd29RclRspStat) -> IfVeSMSuStPassCmprtMd29RclRspStat_Val_write/1
  Subsystem1/36(StPassCmprtMd28RclRspStat) -> IfVeSMSuStPassCmprtMd28RclRspStat_Val_write/1
  Subsystem1/34(StPassCmprtMd26RclRspStat) -> IfVeSMSuStPassCmprtMd26RclRspStat_Val_write/1
  Subsystem1/35(StPassCmprtMd27RclRspStat) -> IfVeSMSuStPassCmprtMd27RclRspStat_Val_write/1
  Subsystem1/33(StPassCmprtMd25RclRspStat) -> IfVeSMSuStPassCmprtMd25RclRspStat_Val_write/1
  Subsystem1/32(StPassCmprtMd24RclRspStat) -> IfVeSMSuStPassCmprtMd24RclRspStat_Val_write/1
  Subsystem1/31(StPassCmprtMd23RclRspStat) -> IfVeSMSuStPassCmprtMd23RclRspStat_Val_write/1
  Subsystem1/30(StPassCmprtMd22RclRspStat) -> IfVeSMSuStPassCmprtMd22RclRspStat_Val_write/1
  Subsystem1/29(StPassCmprtMd21RclRspStat) -> IfVeSMSuStPassCmprtMd21RclRspStat_Val_write/1
  Subsystem1/28(StPassCmprtMd20RclRspStat) -> IfVeSMSuStPassCmprtMd20RclRspStat_Val_write/1
  Subsystem1/27(StPassCmprtMd19RclRspStat) -> IfVeSMSuStPassCmprtMd19RclRspStat_Val_write/1
  Subsystem1/26(StPassCmprtMd18RclRspStat) -> IfVeSMSuStPassCmprtMd18RclRspStat_Val_write/1
  Subsystem1/25(StPassCmprtMd17RclRspStat) -> IfVeSMSuStPassCmprtMd17RclRspStat_Val_write/1
  Subsystem1/24(StPassCmprtMd16RclRspStat) -> IfVeSMSuStPassCmprtMd16RclRspStat_Val_write/1
  Subsystem1/23(StPassCmprtMd15RclRspStat) -> IfVeSMSuStPassCmprtMd15RclRspStat_Val_write/1
  Subsystem1/22(StPassCmprtMd14RclRspStat) -> IfVeSMSuStPassCmprtMd14RclRspStat_Val_write/1
  Subsystem1/21(StPassCmprtMd13RclRspStat) -> IfVeSMSuStPassCmprtMd13RclRspStat_Val_write/1
  Subsystem1/20(StPassCmprtMd12RclRspStat) -> IfVeSMSuStPassCmprtMd12RclRspStat_Val_write/1
  Subsystem1/19(StPassCmprtMd11RclRspStat) -> IfVeSMSuStPassCmprtMd11RclRspStat_Val_write/1
  Subsystem1/18(StPassCmprtMd10RclRspStat) -> IfVeSMSuStPassCmprtMd10RclRspStat_Val_write/1
  Subsystem1/17(StPassCmprtMd9RclRspStat) -> IfVeSMSuStPassCmprtMd9RclRspStat_Val_write/1
  Subsystem1/16(StPassCmprtMd8RclRspStat) -> IfVeSMSuStPassCmprtMd8RclRspStat_Val_write/1
  Subsystem1/15(StPassCmprtMd7RclRspStat) -> IfVeSMSuStPassCmprtMd7RclRspStat_Val_write/1
  Subsystem1/14(StPassCmprtMd6RclRspStat) -> IfVeSMSuStPassCmprtMd6RclRspStat_Val_write/1
  Subsystem1/13(StPassCmprtMd5RclRspStat) -> IfVeSMSuStPassCmprtMd5RclRspStat_Val_write/1
  Subsystem1/12(StPassCmprtMd4RclRspStat) -> IfVeSMSuStPassCmprtMd4RclRspStat_Val_write/1
  Subsystem1/11(StPassCmprtMd3RclRspStat) -> IfVeSMSuStPassCmprtMd3RclRspStat_Val_write/1
  Subsystem1/10(StPassCmprtMd2RclRspStat) -> IfVeSMSuStPassCmprtMd2RclRspStat_Val_write/1
  Subsystem1/9(StPassCmprtMd1RclRspStat) -> IfVeSMSuStPassCmprtMd1RclRspStat_Val_write/1
  Subsystem1/42(StSrv_StMd1_Rsp) -> IfVeSMSuStSrv_StMd1_Rsp_Val_write/1
  Subsystem1/43(StSrv_StMd2_Rsp) -> IfVeSMSuStSrv_StMd2_Rsp_Val_write/1
  Subsystem1/44(StSrv_StMd3_Rsp) -> IfVeSMSuStSrv_StMd3_Rsp_Val_write/1
  Subsystem1/45(StSrv_StMd4_Rsp) -> IfVeSMSuStSrv_StMd4_Rsp_Val_write/1
  Subsystem1/46(StSrv_StMd5_Rsp) -> IfVeSMSuStSrv_StMd5_Rsp_Val_write/1
  Subsystem1/47(StSrv_StMd6_Rsp) -> IfVeSMSuStSrv_StMd6_Rsp_Val_write/1
  Subsystem1/48(StSrv_StMd7_Rsp) -> IfVeSMSuStSrv_StMd7_Rsp_Val_write/1
  Subsystem1/49(StSrv_StMd8_Rsp) -> IfVeSMSuStSrv_StMd8_Rsp_Val_write/1
  Subsystem1/50(StSrv_StMd9_Rsp) -> IfVeSMSuStSrv_StMd9_Rsp_Val_write/1
  Subsystem1/51(StSrv_StMd10_Rsp) -> IfVeSMSuStSrv_StMd10_Rsp_Val_write/1
  Subsystem1/52(StSrv_StMd11_Rsp) -> IfVeSMSuStSrv_StMd11_Rsp_Val_write/1
  Subsystem1/53(StSrv_StMd12_Rsp) -> IfVeSMSuStSrv_StMd12_Rsp_Val_write/1
  Subsystem1/54(StSrv_StMd13_Rsp) -> IfVeSMSuStSrv_StMd13_Rsp_Val_write/1
  Subsystem1/55(StSrv_StMd14_Rsp) -> IfVeSMSuStSrv_StMd14_Rsp_Val_write/1
  Subsystem1/56(StSrv_StMd15_Rsp) -> IfVeSMSuStSrv_StMd15_Rsp_Val_write/1
  Subsystem1/57(StSrv_StMd16_Rsp) -> IfVeSMSuStSrv_StMd16_Rsp_Val_write/1
  Subsystem1/58(StSrv_StMd17_Rsp) -> IfVeSMSuStSrv_StMd17_Rsp_Val_write/1
  Subsystem1/59(StSrv_StMd18_Rsp) -> IfVeSMSuStSrv_StMd18_Rsp_Val_write/1
  Subsystem1/60(StSrv_StMd19_Rsp) -> IfVeSMSuStSrv_StMd19_Rsp_Val_write/1
  Subsystem1/61(StSrv_StMd20_Rsp) -> IfVeSMSuStSrv_StMd20_Rsp_Val_write/1
  Subsystem1/62(StSrv_StMd21_Rsp) -> IfVeSMSuStSrv_StMd21_Rsp_Val_write/1
  Subsystem1/63(StSrv_StMd22_Rsp) -> IfVeSMSuStSrv_StMd22_Rsp_Val_write/1
  Subsystem1/64(StSrv_StMd23_Rsp) -> IfVeSMSuStSrv_StMd23_Rsp_Val_write/1
  Subsystem1/65(StSrv_StMd24_Rsp) -> IfVeSMSuStSrv_StMd24_Rsp_Val_write/1
  Subsystem1/66(StSrv_StMd25_Rsp) -> IfVeSMSuStSrv_StMd25_Rsp_Val_write/1
  Subsystem1/67(StSrv_StMd26_Rsp) -> IfVeSMSuStSrv_StMd26_Rsp_Val_write/1
  Subsystem1/68(StSrv_StMd27_Rsp) -> IfVeSMSuStSrv_StMd27_Rsp_Val_write/1
  Subsystem1/69(StSrv_StMd28_Rsp) -> IfVeSMSuStSrv_StMd28_Rsp_Val_write/1
  Subsystem1/70(StSrv_StMd29_Rsp) -> IfVeSMSuStSrv_StMd29_Rsp_Val_write/1
  Subsystem1/71(StSrv_StMd30_Rsp) -> IfVeSMSuStSrv_StMd30_Rsp_Val_write/1
  Subsystem1/72(StSrv_StMd31_Rsp) -> IfVeSMSuStSrv_StMd31_Rsp_Val_write/1
  Subsystem1/73(StSrv_StMd32_Rsp) -> IfVeSMSuStSrv_StMd32_Rsp_Val_write/1
  isRfFamlyDoneFailed_Val_read/1 -> Subsystem1/82(isFamlyRDoneFailed)
  isRfFamlyDoneOK_Val_read/1 -> Subsystem1/77(isFamlyRDoneOK)
  isLfFamlyDoneOK_Val_read/1 -> Subsystem1/76(isFamlyLDoneOK)
  isINTMDoneOK_Val_read/1 -> Subsystem1/75(isINTMDoneOK)
  isLfLyDoneOK_Val_read/1 -> Subsystem1/78(isLfLyDoneOK)
  isRtLyDoneOK_Val_read/1 -> Subsystem1/79(isRtLyDoneOK)
  isINTMDoneFailed_Val_read/1 -> Subsystem1/80(isINTMDoneFailed)
  isLfFamlyDoneFailed_Val_read/1 -> Subsystem1/81(isFamlyLDoneFailed)
  isLfLyDoneFailed_Val_read/1 -> Subsystem1/83(isLfLyDoneFailed)
  isRtLyDoneFailed_Val_read/1 -> Subsystem1/84(isRtLyDoneFailed)
  isINTMArrivedAtTargetPos_Val_read/1 -> Subsystem1/70(isAcsMdINTMAtTargetPos)
  isLfFamlyArrivedAtTargetPos_Val_read/1 -> Subsystem1/71(isAcsMdFamlyLAtTargetPos)
  isRtFamlyArrivedAtTargetPos_Val_read/1 -> Subsystem1/72(isAcsMdFamlyRAtTargetPos)
  isLfLyArrivedAtTargetPos_Val_read/1 -> Subsystem1/73(isLyLArrivedAtTargetPos)
  isRtLyArrivedAtTargetPos_Val_read/1 -> Subsystem1/74(isLyRArrivedAtTargetPos)
  INTMMdReq_Val_read/1 -> Subsystem1/85(INTMMdReq_Val_read)
  INTMSrcReqTp_Val_read/1 -> Subsystem1/86(INTMSrcReqTp_Val_read)
  LfFamlyReq_Val_read/1 -> Subsystem1/87(LfFamlyReq_Val_read)
  LfFamlySrcReqTp_Val_read/1 -> Subsystem1/88(LfFamlySrcReqTp_Val_read)
  LfLyMdReq_Val_read/1 -> Subsystem1/89(LfLyMdReq_Val_read)
  LfLySrcReqTp_Val_read/1 -> Subsystem1/90(LfLySrcReqTp_Val_read)
  RtFamlyMdReq_Val_read/1 -> Subsystem1/91(RtFamlyMdReq_Val_read)
  RtFamlySrcReqTp_Val_read/1 -> Subsystem1/92(RtFamlySrcReqTp_Val_read)
  RtLyMdReq_Val_read/1 -> Subsystem1/93(RtLyMdReq_Val_read)
  RtLySrcReqTp_Val_read/1 -> Subsystem1/94(RtLySrcReqTp_Val_read)
  SoftIntINTM_Val_read/1 -> Subsystem1/95(SoftIntINTM_Val_read)
  SoftIntLfFamly_Val_read/1 -> Subsystem1/96(SoftIntLfFamly_Val_read)
  SoftIntLfLy_Val_read/1 -> Subsystem1/97(SoftIntLfLy_Val_read)
  SoftIntRtFamly_Val_read/1 -> Subsystem1/98(SoftIntRtFamly_Val_read)
  SwIntRtLy_Val_read/1 -> Subsystem1/104(SwIntRtLy_Val_read)
  SoftIntRtLy_Val_read/1 -> Subsystem1/99(SoftIntRtLy_Val_read)
  SwIntINTM_Val_read/1 -> Subsystem1/100(SwIntINTM_Val_read)
  SwIntLfFamly_Val_read/1 -> Subsystem1/101(SwIntLfFamly_Val_read)
  SwIntLfLy_Val_read/1 -> Subsystem1/102(SwIntLfLy_Val_read)
  SwIntRtFamly_Val_read/1 -> Subsystem1/103(SwIntRtFamly_Val_read)
  PosArray_Val_read/1 -> Subsystem1/105(PosArray_Val_read)
  AllVipSrcReqTp_Val_read/1 -> Subsystem1/106(AllVipSrcReqTp_Val_read)
  LugMdLtAvl_Val_read/1 -> Subsystem1/107(LugMdLtAvl_Val_read)
  LugMdRtAvl_Val_read/1 -> Subsystem1/108(LugMdRtAvl_Val_read)
  VipMdLtAvl_Val_read/1 -> Subsystem1/109(VipMdLtAvl_Val_read)
  VipMdRtAvl_Val_read/1 -> Subsystem1/110(VipMdRtAvl_Val_read)
  SwIntAllVip_Val_read/1 -> Subsystem1/111(SwIntAllVip_Val_read)
  isLgrstCloseRArrivedAtTargetPos_Val_read/1 -> Subsystem1/120(isLgrstCloseRArrivedAtTargetPos_Val_read)
  isLgrstCloseRDoneFailed_Val_read/1 -> Subsystem1/121(isLgrstCloseRDoneFailed_Val_read)
  isLgrstCloseLArrivedAtTargetPos_Val_read/1 -> Subsystem1/117(isLgrstCloseLArrivedAtTargetPos_Val_read)
  isLgrstCloseLDoneFailed_Val_read/1 -> Subsystem1/118(isLgrstCloseLDoneFailed_Val_read)
  isLgrstCloseLDoneOK_Val_read/1 -> Subsystem1/119(isLgrstCloseLDoneOK_Val_read)
  isLgrstCloseRDoneOK_Val_read/1 -> Subsystem1/122(isLgrstCloseRDoneOK_Val_read)
  isLgrstOpenLArrivedAtTargetPos_Val_read/1 -> Subsystem1/123(isLgrstOpenLArrivedAtTargetPos_Val_read)
  isLgrstOpenLDoneFailed_Val_read/1 -> Subsystem1/124(isLgrstOpenLDoneFailed_Val_read)
  isINTMRDoneFailed_Val_read/1 -> Subsystem1/115(isINTMRDoneFailed_Val_read)
  isINTMRDoneOK_Val_read/1 -> Subsystem1/116(isINTMRDoneOK_Val_read)
  isLgrstOpenLDoneOK_Val_read/1 -> Subsystem1/125(isLgrstOpenLDoneOK_Val_read)
  isLgrstOpenRArrivedAtTargetPos_Val_read/1 -> Subsystem1/126(isLgrstOpenRArrivedAtTargetPos_Val_read)
  IntimacyRtMdReq_Val_read/1 -> Subsystem1/112(IntimacyRtMdReq_Val_read)
  IntimacyRtMdSrcTp_Val_read/1 -> Subsystem1/113(IntimacyRtMdSrcTp_Val_read)
  isINTMRArrivedAtTargetPos_Val_read/1 -> Subsystem1/114(isINTMRArrivedAtTargetPos_Val_read)
  isLgrstOpenRDoneFailed_Val_read/1 -> Subsystem1/127(isLgrstOpenRDoneFailed_Val_read)
  isLgrstOpenRDoneOK_Val_read/1 -> Subsystem1/128(isLgrstOpenRDoneOK_Val_read)
  LgrstCloseLtMdReq_Val_read/1 -> Subsystem1/129(LgrstCloseLtMdReq_Val_read)
  LgrstCloseLtSrcReqTp_Val_read/1 -> Subsystem1/130(LgrstCloseLtSrcReqTp_Val_read)
  LgrstCloseRtMdReq_Val_read/1 -> Subsystem1/131(LgrstCloseRtMdReq_Val_read)
  LgrstCloseRtSrcReqTp_Val_read/1 -> Subsystem1/132(LgrstCloseRtSrcReqTp_Val_read)
  LgrstOpenLtMdReq_Val_read/1 -> Subsystem1/133(LgrstOpenLtMdReq_Val_read)
  LgrstOpenLtSrcReqTp_Val_read/1 -> Subsystem1/134(LgrstOpenLtSrcReqTp_Val_read)
  LgrstOpenRtMdReq_Val_read/1 -> Subsystem1/135(LgrstOpenRtMdReq_Val_read)
  LgrstOpenRtSrcReqTp_Val_read/1 -> Subsystem1/136(LgrstOpenRtSrcReqTp_Val_read)
  SoftIntIntimacyRt_Val_read/1 -> Subsystem1/137(SoftIntIntimacyRt_Val_read)
  SoftIntLgrstCloseLt_Val_read/1 -> Subsystem1/138(SoftIntLgrstCloseLt_Val_read)
  SoftIntLgrstCloseRt_Val_read/1 -> Subsystem1/139(SoftIntLgrstCloseRt_Val_read)
  SoftIntLgrstOpenLt_Val_read/1 -> Subsystem1/140(SoftIntLgrstOpenLt_Val_read)
  SoftIntLgrstOpenRt_Val_read/1 -> Subsystem1/141(SoftIntLgrstOpenRt_Val_read)
  SwIntIntimacyRt_Val_read/1 -> Subsystem1/142(SwIntIntimacyRt_Val_read)
  SwIntLgrstCloseLt_Val_read/1 -> Subsystem1/143(SwIntLgrstCloseLt_Val_read)
  SwIntLgrstCloseRt_Val_read/1 -> Subsystem1/144(SwIntLgrstCloseRt_Val_read)
  SwIntLgrstOpenLt_Val_read/1 -> Subsystem1/145(SwIntLgrstOpenLt_Val_read)
  SwIntLgrstOpenRt_Val_read/1 -> Subsystem1/146(SwIntLgrstOpenRt_Val_read)
